simulink model "Lab2"  (R2021b)
settings: Solver=VariableStepAuto  StartTime=0.0  StopTime=40.0  RelTol=1e-3
values from neighbouring files (symbols this model uses):
  Hd1 = c2d(H, Ts2, 'zoh')    [Lab1.m]    (also in Lab2.m = c2d(Hcpi, Ts1, 'zoh'))
  Hd2 = c2d(H, Ts2, 'tustin')    [Lab1.m]    (also in Lab2.m = c2d(Hcpd, Ts2, 'zoh'))
  Ts1 = 1    [Lab1.m]    (also in Lab2.m = 6)
  Ts2 = 2    [Lab1.m]    (also in Lab2.m = 1.8)
settings Model: Creator=User  LastModifiedBy=User

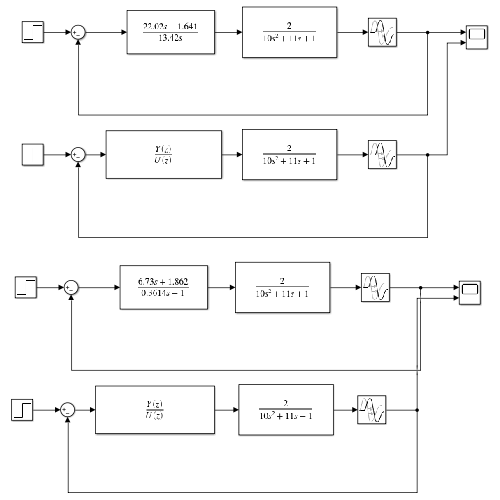
[thumbnail: Simulink's stored preview of the top-level diagram]
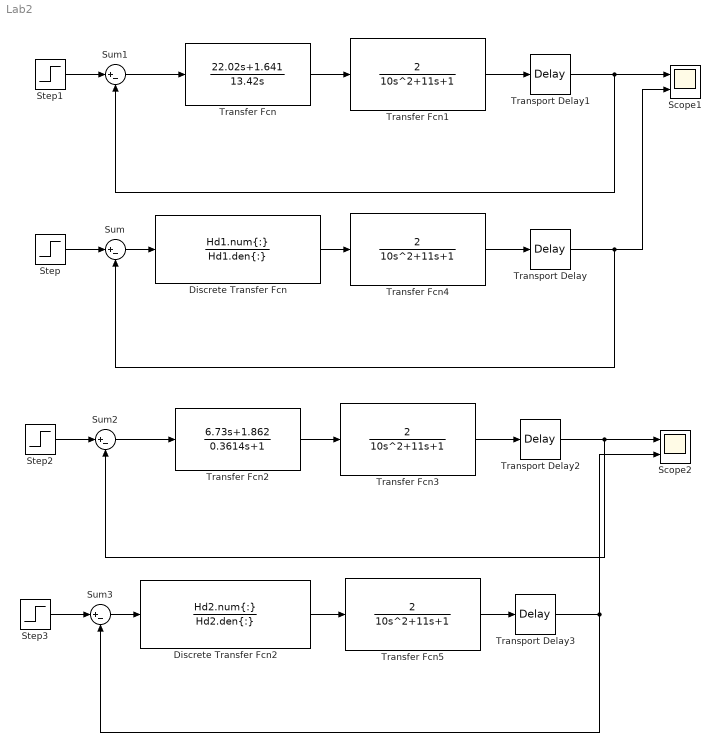
== system Lab2 ==
  Discrete Transfer Fcn : DiscreteTransferFcn  Numerator=Hd1.num{:}  Denominator=Hd1.den{:}  SampleTime=Ts1
  Discrete Transfer Fcn2 : DiscreteTransferFcn  Numerator=Hd2.num{:}  Denominator=Hd2.den{:}  SampleTime=Ts2
  Scope1 : Scope  NumInputPorts=2
  Scope2 : Scope  NumInputPorts=2
  Step{,1..3} (4 alike) : Step  Before=1  SampleTime=0
  Sum{,1..3} (4 alike) : Sum  Inputs=|+-
  Transfer Fcn : TransferFcn  Numerator=[22.02 1.641]  Denominator=[13.42 0]
  Transfer Fcn{1,3..5} (4 alike) : TransferFcn  Numerator=[2]  Denominator=[10 11 1]
  Transfer Fcn2 : TransferFcn  Numerator=[6.73 1.862]  Denominator=[0.3614 1]
  Transport Delay{,1..3} (4 alike) : TransportDelay
  wires:
  Step/1 -> Sum/1
  Sum/1 -> Discrete Transfer Fcn/1
  Transport Delay/1 -> Scope1/2, Sum/2
  Transport Delay1/1 -> Sum1/2, Scope1/1
  Step1/1 -> Sum1/1
  Sum1/1 -> Transfer Fcn/1
  Transfer Fcn/1 -> Transfer Fcn1/1
  Transfer Fcn1/1 -> Transport Delay1/1
  Transport Delay2/1 -> Sum2/2, Scope2/1
  Transfer Fcn2/1 -> Transfer Fcn3/1
  Step2/1 -> Sum2/1
  Sum2/1 -> Transfer Fcn2/1
  Transfer Fcn3/1 -> Transport Delay2/1
  Transfer Fcn5/1 -> Transport Delay3/1
  Transport Delay3/1 -> Scope2/2, Sum3/2
  Discrete Transfer Fcn2/1 -> Transfer Fcn5/1
  Step3/1 -> Sum3/1
  Sum3/1 -> Discrete Transfer Fcn2/1
  Discrete Transfer Fcn/1 -> Transfer Fcn4/1
  Transfer Fcn4/1 -> Transport Delay/1
